simulink model "simulacion1"  (R2025a)
settings: Solver=ode8  StartTime=0.0  StopTime=40  FixedStep=0.01  RelTol=1e-3
settings Model: Creator=440G5  LastModifiedBy=440G5

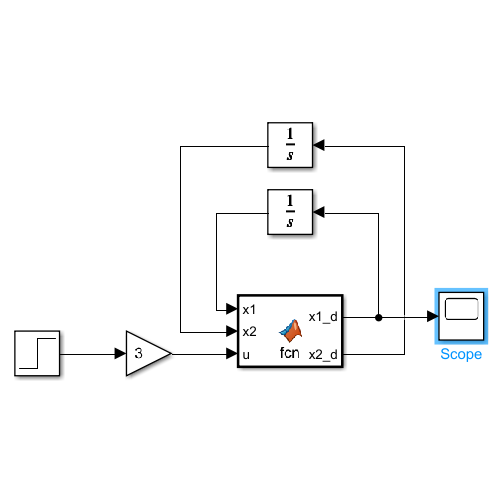
[thumbnail: Simulink's stored preview of the top-level diagram]
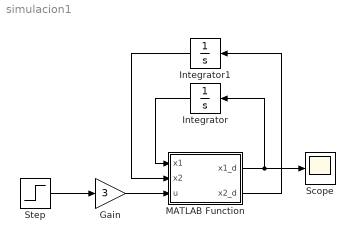
== system simulacion1 ==
  Gain : Gain  Gain=3
  Integrator : Integrator
  Integrator1 : Integrator
  MATLAB Function : MATLAB Function  TreatAsAtomicUnit=on
  Scope : Scope
      settings: ActiveDisplayYMinimum=-8.045646558136152  ActiveDisplayYMaximum=10.591841064009039
  Step : Step  SampleTime=0
  wires:
  MATLAB Function/1(x1_d) -> Scope/1, Integrator/1
  Integrator/1 -> MATLAB Function/1(x1)
  MATLAB Function/2(x2_d) -> Integrator1/1
  Integrator1/1 -> MATLAB Function/2(x2)
  Step/1 -> Gain/1
  Gain/1 -> MATLAB Function/3(u)

== matlab function simulacion1/MATLAB Function ==
  data: x1 input; x2 input; u input; x1_d output; x2_d output
function [x1_d, x2_d] = fcn(x1, x2, u)

l = 0.5;
m = 0.5;
g = 9.81;
b = 0.4;

x1_d = x2;
x2_d = (g/l)*sin(x1) -(b/m*l)*x2 + u/m*l*l;
